simulink model "Feedforward_template"  (R2020a)
settings: Solver=VariableStepAuto  StartTime=0.0  StopTime=60  RelTol=1e-3
libraries: simulink x4
settings Model: Creator=David Wiman  LastModifiedBy=David Wiman

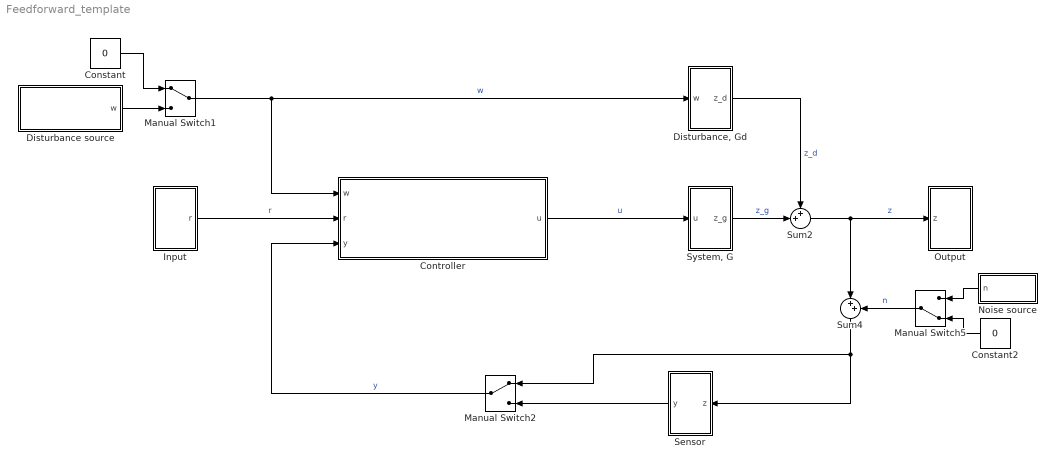
== system Feedforward_template ==
  Constant : Constant  Value=0
  Constant2 : Constant  Value=0
  Controller : Subsystem
  Disturbance source : Subsystem
  "Disturbance, Gd" : Subsystem
  Input : Subsystem
  Manual Switch1 : ManualSwitch
  Manual Switch2 : ManualSwitch
  Manual Switch5 : ManualSwitch  CurrentSetting=0
  Noise source : Subsystem
  Output : Subsystem
  Sensor : Subsystem
  Sum2 : Sum  Inputs=++|
  Sum4 : Sum  Inputs=|++
  "System, G" : Subsystem
  wires:
  Constant/1 -> Manual Switch1/1
  Manual Switch1/1 -> Controller/1(w), "Disturbance, Gd"/1(w)  "w"
  Sum2/1 -> Output/1(z), Sum4/1  "z"
  "Disturbance, Gd"/1(z_d) -> Sum2/1  "z_d"
  "System, G"/1(z_g) -> Sum2/2  "z_g"
  Sensor/1(y) -> Manual Switch2/2
  Disturbance source/1(w) -> Manual Switch1/2
  Sum4/1 -> Manual Switch2/1, Sensor/1(z)
  Manual Switch5/1 -> Sum4/2  "n"
  Constant2/1 -> Manual Switch5/2
  Noise source/1(n) -> Manual Switch5/1
  Input/1(r) -> Controller/2(r)  "r"
  Manual Switch2/1 -> Controller/3(y)  "y"
  Controller/1(u) -> "System, G"/1(u)  "u"

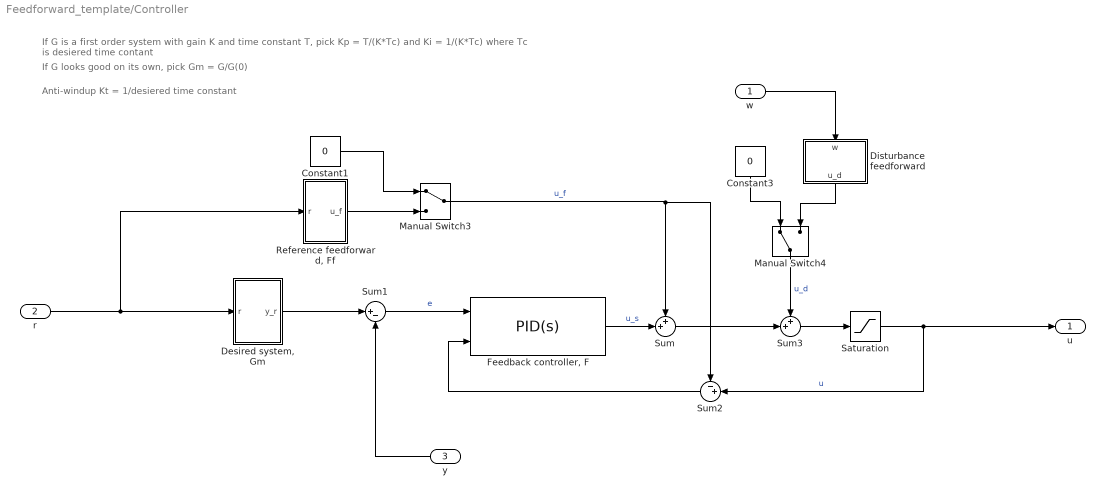
== system Feedforward_template/Controller ==
  note: Anti-windup Kt = 1/desiered time constant
  note: If G looks good on its own, pick Gm = G/G(0)
  note: If G is a first order system with gain K and time constant T, pick Kp = T/(K*Tc) and Ki = 1/(K*Tc) where Tc is desiered time contant
  w : Inport
  r : Inport  Port=2
  y : Inport  Port=3
  Constant1 : Constant  Value=0
  Constant3 : Constant  Value=0
  "Desired system, Gm" : Subsystem
  Disturbance feedforward : Subsystem
  "Feedback controller, F" : simulink/Continuous/PID Controller  Controller=PID  Form=Parallel  TimeDomain=Continuous-time  UseExternalTs=off  SampleTime=-1  IntegratorMethod=Forward Euler  FilterMethod=Forward Euler  ControllerParametersSource=internal  P=5  I=2  D=7  UseFilter=on  N=100  TunerSelectOption=Transfer Function Based (PID Tuner App)  InitialConditionSource=internal  InitialConditionForIntegrator=0  InitialConditionForFilter=0  DifferentiatorICPrevScaledInput=0  ExternalReset=none  TrackingMode=on  Kt=1  LimitOutput=off  UpperSaturationLimit=inf  LowerSaturationLimit=-inf  LinearizeAsGain=on  AntiWindupMode=none  Kb=1  POutMin=[]  POutMax=[]  IOutMin=[]  IOutMax=[]  DOutMin=[]  DOutMax=[]  NOutMin=[]  NOutMax=[]  SumOutMin=[]  SumOutMax=[]  SaturationOutMin=[]  SaturationOutMax=[]  PParamMin=[]  PParamMax=[]  IParamMin=[]  IParamMax=[]  DParamMin=[]  DParamMax=[]  NParamMin=[]  NParamMax=[]  KbParamMin=[]  KbParamMax=[]  KtParamMin=[]  KtParamMax=[]  KbOutMin=[]  KbOutMax=[]  KtOutMin=[]  KtOutMax=[]  IntegratorOutMin=[]  IntegratorOutMax=[]  FilterOutMin=[]  FilterOutMax=[]  SumI1OutMin=[]  SumI1OutMax=[]  SumI2OutMin=[]  SumI2OutMax=[]  SumI3OutMin=[]  SumI3OutMax=[]  SumI4OutMin=[]  SumI4OutMax=[]  SumDOutMin=[]  SumDOutMax=[]  DifferentiatorOutMin=[]  DifferentiatorOutMax=[]  FilterDiffOutCoefMin=[]  FilterDiffOutCoefMax=[]  ReciprocalOutMin=[]  ReciprocalOutMax=[]  SumDenOutMin=[]  SumDenOutMax=[]  SumNumOutMin=[]  SumNumOutMax=[]  DivideOutMin=[]  DivideOutMax=[]  UdiffTsProdOutMin=[]  UdiffTsProdOutMax=[]  NTsProdOutMin=[]  NTsProdOutMax=[]  UintegralTsProdOutMin=[]  UintegralTsProdOutMax=[]  UngainTsProdOutMin=[]  UngainTsProdOutMax=[]  IntegratorContinuousStateAttributes=''  IntegratorStateMustResolveToSignalObject=off  IntegratorRTWStateStorageClass=Auto  FilterContinuousStateAttributes=''  FilterStateMustResolveToSignalObject=off  FilterRTWStateStorageClass=Auto  ParallelPVariant=InternalParameters  IdealPVariant=Disabled  IVariant=InternalParameters  DVariant=InternalParameters  IntegratorVariant=Continuous  SatVariant=Disabled  AWVariant=Passthrough  PCopyVariant=Disabled  TRVariant=Enabled  FdbkBlocksVariant=Forward  IdealPFdbkVariant=Disabled  SatFdbkVariant=Disabled  DerivativeFilterVariant=ContFilter  NVariant=InternalParameters  NCopyVariant=Disabled  FilterICVariant=InternalICsFilter  IntegratorICVariant=InternalICs  ExternalResetVariant=Disabled  TRSumVariant=TrackingMode  SumFdbkVariant=Disabled  SumVariant=Sum_PID  TsampFilterVariant=InternalTs  TsampNgainVariant=Passthrough  TsampIntegralVariant=Passthrough
  Manual Switch3 : ManualSwitch
  Manual Switch4 : ManualSwitch
  "Reference feedforward, Ff" : Subsystem
  Saturation : Saturate  UpperLimit=10
  Sum : Sum  Inputs=++|
  Sum1 : Sum  Inputs=|+-
  Sum2 : Sum  Inputs=-+|
  Sum3 : Sum  Inputs=++|
  u : Outport
  wires:
  Constant3/1 -> Manual Switch4/1
  Sum1/1 -> "Feedback controller, F"/1  "e"
  "Desired system, Gm"/1(y_r) -> Sum1/1
  "Feedback controller, F"/1 -> Sum/2  "u_s"
  Disturbance feedforward/1(u_d) -> Manual Switch4/2
  y/1 -> Sum1/2
  Manual Switch3/1 -> Sum2/1, Sum/1  "u_f"
  r/1 -> "Desired system, Gm"/1(r), "Reference feedforward, Ff"/1(r)
  Manual Switch4/1 -> Sum3/1  "u_d"
  Sum3/1 -> Saturation/1
  Constant1/1 -> Manual Switch3/1
  "Reference feedforward, Ff"/1(u_f) -> Manual Switch3/2
  Sum/1 -> Sum3/2
  w/1 -> Disturbance feedforward/1(w)
  Saturation/1 -> u/1, Sum2/2  "u"
  Sum2/1 -> "Feedback controller, F"/2

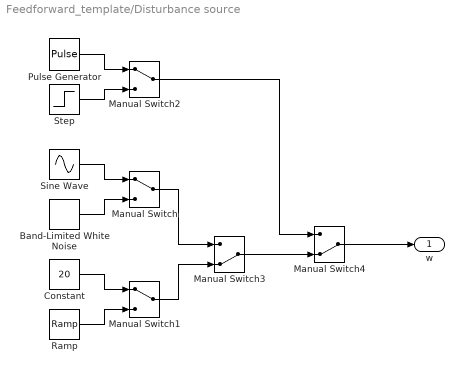
== system Feedforward_template/Disturbance source ==
  Band-Limited White Noise : simulink/Sources/Band-Limited White Noise  Cov=[0.1]  Ts=0.1  seed=[23341]
  Constant : Constant  Value=20
  Manual Switch : ManualSwitch
  Manual Switch1 : ManualSwitch
  Manual Switch2 : ManualSwitch
  Manual Switch3 : ManualSwitch  CurrentSetting=0
  Manual Switch4 : ManualSwitch  CurrentSetting=0
  Pulse Generator : DiscretePulseGenerator  PulseType=Time based  Period=10  PulseWidth=5
  Ramp : simulink/Sources/Ramp  slope=1  start=0  InitialOutput=0
  Sine Wave : Sin  SampleTime=0
  Step : Step  SampleTime=0
  w : Outport
  wires:
  Step/1 -> Manual Switch2/2
  Pulse Generator/1 -> Manual Switch2/1
  Sine Wave/1 -> Manual Switch/1
  Band-Limited White Noise/1 -> Manual Switch/2
  Constant/1 -> Manual Switch1/1
  Ramp/1 -> Manual Switch1/2
  Manual Switch/1 -> Manual Switch3/1
  Manual Switch1/1 -> Manual Switch3/2
  Manual Switch3/1 -> Manual Switch4/2
  Manual Switch2/1 -> Manual Switch4/1
  Manual Switch4/1 -> w/1

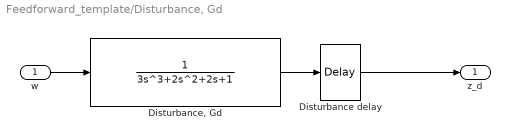
== system Feedforward_template/Disturbance, Gd ==
  w : Inport
  Disturbance delay : TransportDelay  DelayTime=0
  "Disturbance, Gd" : TransferFcn  Denominator=[3 2 2 1]
  z_d : Outport
  wires:
  "Disturbance, Gd"/1 -> Disturbance delay/1
  Disturbance delay/1 -> z_d/1
  w/1 -> "Disturbance, Gd"/1

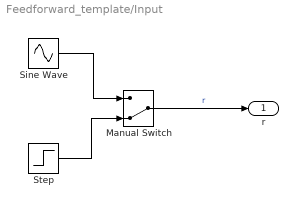
== system Feedforward_template/Input ==
  Manual Switch : ManualSwitch  CurrentSetting=0
  Sine Wave : Sin  Amplitude=10  Bias=20  SampleTime=0
  Step : Step  Time=10  After=20  SampleTime=0
  r : Outport
  wires:
  Step/1 -> Manual Switch/2
  Sine Wave/1 -> Manual Switch/1
  Manual Switch/1 -> r/1  "r"

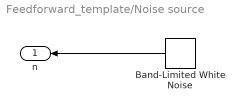
== system Feedforward_template/Noise source ==
  Band-Limited White Noise : simulink/Sources/Band-Limited White Noise  Cov=[0.1]  Ts=0.1  seed=[23341]
  n : Outport
  wires:
  Band-Limited White Noise/1 -> n/1

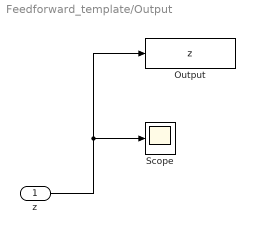
== system Feedforward_template/Output ==
  z : Inport
  Output : ToWorkspace  VariableName=z  SampleTime=-1
  Scope : Scope
  wires:
  z/1 -> Scope/1, Output/1

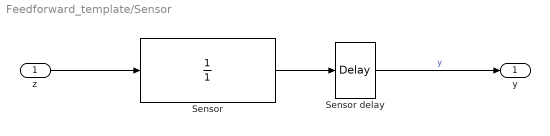
== system Feedforward_template/Sensor ==
  z : Inport
  Sensor : TransferFcn  Denominator=[1]
  Sensor delay : TransportDelay  DelayTime=0
  y : Outport
  wires:
  Sensor delay/1 -> y/1  "y"
  Sensor/1 -> Sensor delay/1
  z/1 -> Sensor/1

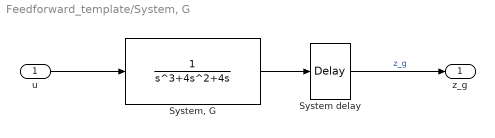
== system Feedforward_template/System, G ==
  u : Inport
  System delay : TransportDelay  DelayTime=0
  "System, G" : TransferFcn  Denominator=[1 4 4 0]
  z_g : Outport
  wires:
  "System, G"/1 -> System delay/1
  System delay/1 -> z_g/1  "z_g"
  u/1 -> "System, G"/1

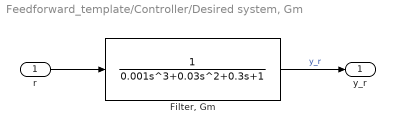
== system Feedforward_template/Controller/Desired system, Gm ==
  r : Inport
  "Filter, Gm" : TransferFcn  Denominator=[0.001 0.03 0.3 1]
  y_r : Outport
  wires:
  r/1 -> "Filter, Gm"/1
  "Filter, Gm"/1 -> y_r/1  "y_r"

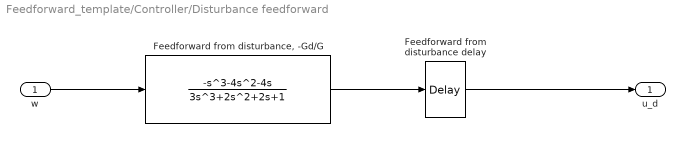
== system Feedforward_template/Controller/Disturbance feedforward ==
  w : Inport
  "Feedforward from disturbance delay " : TransportDelay  DelayTime=0
  "Feedforward from disturbance, -Gd/G" : TransferFcn  Numerator=[-1 -4 -4 0]  Denominator=[3 2 2 1]
  u_d : Outport
  wires:
  "Feedforward from disturbance, -Gd/G"/1 -> "Feedforward from disturbance delay "/1
  "Feedforward from disturbance delay "/1 -> u_d/1
  w/1 -> "Feedforward from disturbance, -Gd/G"/1

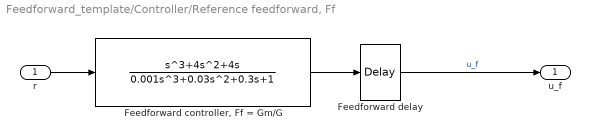
== system Feedforward_template/Controller/Reference feedforward, Ff ==
  r : Inport
  "Feedforward controller, Ff = Gm/G " : TransferFcn  Numerator=[1 4 4 0]  Denominator=[0.001 0.03 0.3 1]
  Feedforward delay : TransportDelay  DelayTime=0
  u_f : Outport
  wires:
  "Feedforward controller, Ff = Gm/G "/1 -> Feedforward delay/1
  r/1 -> "Feedforward controller, Ff = Gm/G "/1
  Feedforward delay/1 -> u_f/1  "u_f"
